simulink model "First_order_simulink"  (R2020b)
settings: Solver=VariableStepAuto  StartTime=0.0  StopTime=100  RelTol=1e-3
settings Model: Creator=99003785  LastModifiedBy=99003785

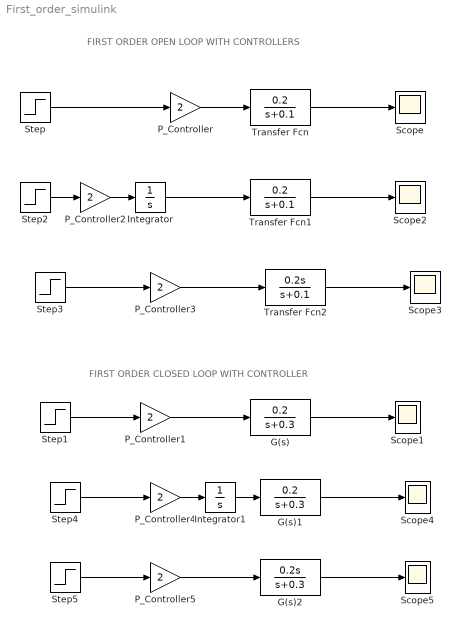
== system First_order_simulink ==
  note: FIRST ORDER OPEN LOOP WITH CONTROLLERS
  note: FIRST ORDER CLOSED LOOP WITH CONTROLLER
  G(s) : TransferFcn  Numerator=[0.2]  Denominator=[1 0.3]
  G(s)1 : TransferFcn  Numerator=[0.2]  Denominator=[1 0.3]
  G(s)2 : TransferFcn  Numerator=[0.2,0]  Denominator=[1 0.3]
  Integrator : Integrator
  Integrator1 : Integrator
  P_Controller{,1..5} (6 alike) : Gain  Gain=2
  Scope{,1..5} (6 alike) : Scope
  Step{,1..5} (6 alike) : Step  SampleTime=0
  Transfer Fcn : TransferFcn  Numerator=[0.2]  Denominator=[1 0.1]
  Transfer Fcn1 : TransferFcn  Numerator=[0.2]  Denominator=[1 0.1]
  Transfer Fcn2 : TransferFcn  Numerator=[0.2,0]  Denominator=[1 0.1]
  wires:
  Transfer Fcn/1 -> Scope/1
  P_Controller/1 -> Transfer Fcn/1
  Step/1 -> P_Controller/1
  G(s)/1 -> Scope1/1
  Step1/1 -> P_Controller1/1
  P_Controller1/1 -> G(s)/1
  Transfer Fcn1/1 -> Scope2/1
  Integrator/1 -> Transfer Fcn1/1
  Step2/1 -> P_Controller2/1
  P_Controller2/1 -> Integrator/1
  Transfer Fcn2/1 -> Scope3/1
  Step3/1 -> P_Controller3/1
  P_Controller3/1 -> Transfer Fcn2/1
  G(s)1/1 -> Scope4/1
  Step4/1 -> P_Controller4/1
  P_Controller4/1 -> Integrator1/1
  Integrator1/1 -> G(s)1/1
  G(s)2/1 -> Scope5/1
  P_Controller5/1 -> G(s)2/1
  Step5/1 -> P_Controller5/1
